simulink model "motor_discrete_velocity"  (R2015b)
settings: Solver=VariableStepAuto  StartTime=0.0  StopTime=simtime  RelTol=1e-3
values from neighbouring files (symbols this model uses):
  D = [0 0; 0 0; 0 0]    [Velocity_ctrl_HYDRAULIC.m]    (also in ex1.m = 0; position_ctrl.m = 0; velocity_ctrl.m = 0)
  d_v = 1    [ex1.m]    (also in motor_parameters.mat; position_ctrl.m; velocity_ctrl.m)
  enable_karnop = 0    [discrete_velocity.m]    (also in ex1.m = 1; motor_parameters.mat = 1; pcontrol.m; pcontrol_position.m)
  enable_sin = 0    [discrete_velocity.m]    (also in ex1.m = 1; motor_parameters.mat; pcontrol.m = 1; pcontrol_position.m = 1)
  F_c = 1e-3    (= 0.001)    [ex1.m]    (also in motor_parameters.mat; position_ctrl.m; velocity_ctrl.m)
  I = 1    [ex1.m]    (also in pcontrol.m = 0; pcontrol_position.m = 0; picontroller.m = omega1*omega2*n*Jtot*m.R/m.k; position_ctrl.m = 2)
  J = J1+J2    (= 3.6e-05)    [ex1.m]    (also in lec_example.m = 0.1; position_ctrl.m; velocity_ctrl.m)
  motor = motor_pars    [ex1.m]    (also in position_ctrl.m; velocity_ctrl.m)
  n = 5    [ex1.m]    (also in motor_parameters.mat; position_ctrl.m; velocity_ctrl.m)
  P = 0.5    [Velocity_ctrl_HYDRAULIC.m]    (also in ex1.m = 20; pcontrol.m = 8; pcontrol_position.m = 4; picontroller.m = n*(Jtot*omega1*m.R+Jtot*omega2*m.R-m.d*m.R-m.k^2)/m.k)
  sim_sin_amp = 200    [ex1.m]    (also in motor_parameters.mat = 1; pcontrol.m = 10; pcontrol_position.m = 10; pdcontroller_position.m = 10)
  sim_sin_freq = 10    [ex1.m]    (also in motor_parameters.mat = 1; pcontrol.m = 1; pcontrol_position.m = 1; pdcontroller_position.m = 1)
  sim_v = Vmax    (= 24)    [ex1.m]    (also in motor_parameters.mat; pcontrol.m = 1; pcontrol_position.m = 1; pdcontroller_position.m = 1)
  sim_zoh = 0.02    [discrete_velocity.m]    (also in pcontrol.m = 0.002; pcontrol_position.m; pdcontroller_position.m = 0.002; picontroller.m = 0.002)
  sim_zoh_sample_time = zoh_sample_time*1e-3    (= 2e-06)    [discrete_velocity.m]    (also in ex1.m = 0; motor_parameters.mat = 0; position_ctrl.m; velocity_ctrl.m)
libraries: simulink x3
settings Model: Creator=Gabriel  LastModifiedBy=Gabriel

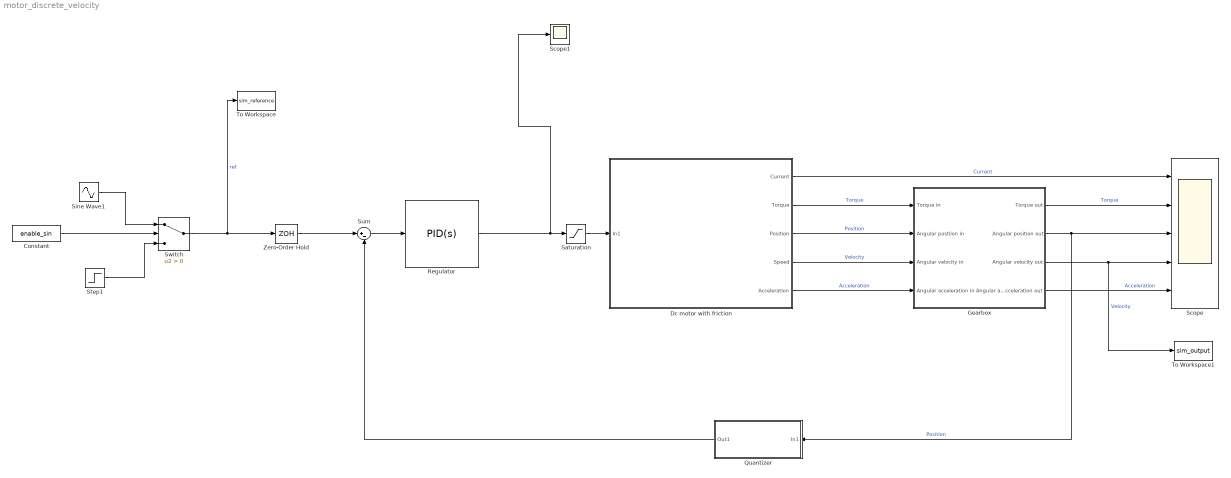
== system motor_discrete_velocity ==
  Constant : Constant  Value=enable_sin
  Dc motor with friction : Subsystem
      mask Display:
      | image('dcmotor.jpg')
      | port_label('input', 1, 'Voltage')
      | port_label('output', 1, 'Current')
      | port_label('output', 2, 'Torque')
      | port_label('output', 3, 'Position')
      | port_label('output', 4, 'Velocity')
      | port_label('output', 5, 'Acceleration')
  Gearbox : Subsystem
  "Quantizer " : Subsystem
  Regulator : simulink/Continuous/PID Controller  Controller=PID  TimeDomain=Continuous-time  SampleTime=-1  IntegratorMethod=Forward Euler  FilterMethod=Forward Euler  Form=Parallel  UseFilter=on  ControllerParametersSource=internal  P=P  I=I  D=D  N=100  InitialConditionSource=internal  InitialConditionForIntegrator=0  InitialConditionForFilter=0  ExternalReset=none  LimitOutput=off  UpperSaturationLimit=inf  LowerSaturationLimit=-inf  LinearizeAsGain=on  AntiWindupMode=none  Kb=1  TrackingMode=off  Kt=1  PParamMin=[]  PParamMax=[]  IParamMin=[]  IParamMax=[]  DParamMin=[]  DParamMax=[]  NParamMin=[]  NParamMax=[]  KbParamMin=[]  KbParamMax=[]  KtParamMin=[]  KtParamMax=[]  POutMin=[]  POutMax=[]  IOutMin=[]  IOutMax=[]  DOutMin=[]  DOutMax=[]  NOutMin=[]  NOutMax=[]  KbOutMin=[]  KbOutMax=[]  KtOutMin=[]  KtOutMax=[]  IntegratorOutMin=[]  IntegratorOutMax=[]  FilterOutMin=[]  FilterOutMax=[]  SumOutMin=[]  SumOutMax=[]  SumI1OutMin=[]  SumI1OutMax=[]  SumI2OutMin=[]  SumI2OutMax=[]  SumI3OutMin=[]  SumI3OutMax=[]  SumDOutMin=[]  SumDOutMax=[]  SaturationOutMin=[]  SaturationOutMax=[]  IntegratorContinuousStateAttributes=''  IntegratorStateMustResolveToSignalObject=off  IntegratorRTWStateStorageClass=Auto  FilterContinuousStateAttributes=''  FilterStateMustResolveToSignalObject=off  FilterRTWStateStorageClass=Auto  DifferentiatorICPrevScaledInput=0  DifferentiatorOutMin=[]  DifferentiatorOutMax=[]
  Saturation : Saturate  UpperLimit=24  LowerLimit=-24
  Scope : Scope  NumInputPorts=5
  Scope1 : Scope
  Sine Wave1 : Sin  Amplitude=sim_sin_amp  Frequency=sim_sin_freq  SampleTime=0
  Step1 : Step  Time=0  After=sim_v  SampleTime=0
  Sum : Sum  Inputs=|+-
  Switch : Switch  Criteria=u2 > Threshold
  To Workspace : ToWorkspace  VariableName=sim_reference  SaveFormat=Timeseries  SampleTime=-1
  To Workspace1 : ToWorkspace  VariableName=sim_output  SaveFormat=Timeseries  SampleTime=-1
  Zero-Order Hold : ZeroOrderHold  SampleTime=sim_zoh
  wires:
  Sum/1 -> Regulator/1
  Zero-Order Hold/1 -> Sum/1
  Step1/1 -> Switch/3
  Sine Wave1/1 -> Switch/1
  Constant/1 -> Switch/2
  Switch/1 -> Zero-Order Hold/1, To Workspace/1  "ref"
  Dc motor with friction/4(Speed) -> Gearbox/3(Angular velocity in)  "Velocity"
  Dc motor with friction/2(Torque) -> Gearbox/1(Torque in)  "Torque"
  Dc motor with friction/1(Current) -> Scope/1  "Current"
  Dc motor with friction/5(Acceleration) -> Gearbox/4(Angular acceleration in)  "Acceleration"
  Dc motor with friction/3(Position) -> Gearbox/2(Angular postiion in)  "Position"
  Gearbox/1(Torque out) -> Scope/2  "Torque"
  Gearbox/2(Angular position out) -> "Quantizer "/1(In1), Scope/3  "Position"
  Gearbox/3(Angular velocity out) -> To Workspace1/1, Scope/4  "Velocity"
  Gearbox/4(Angular acceleration out) -> Scope/5  "Acceleration"
  Regulator/1 -> Saturation/1, Scope1/1
  "Quantizer "/1(Out1) -> Sum/2
  Saturation/1 -> Dc motor with friction/1(In1)

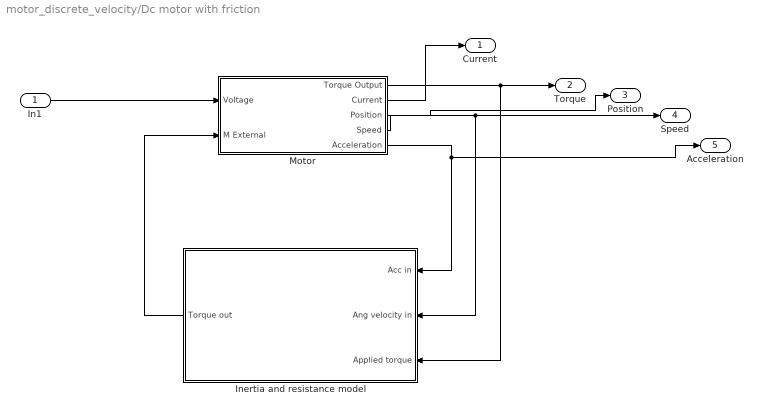
== system motor_discrete_velocity/Dc motor with friction ==
  In1 : Inport
  "Inertia and resistance model " : Subsystem
  Motor : Subsystem
  Current : Outport
  Torque : Outport  Port=2
  Position : Outport  Port=3
  Speed : Outport  Port=4
  Acceleration : Outport  Port=5
  wires:
  Motor/4(Speed) -> Speed/1, "Inertia and resistance model "/2(Ang velocity in)
  Motor/3(Position) -> Position/1
  Motor/2(Current) -> Current/1
  "Inertia and resistance model "/1(Torque out) -> Motor/2("M External ")
  Motor/1(Torque Output) -> Torque/1, "Inertia and resistance model "/3(Applied torque)
  In1/1 -> Motor/1(Voltage)
  Motor/5(Acceleration) -> "Inertia and resistance model "/1(Acc in), Acceleration/1

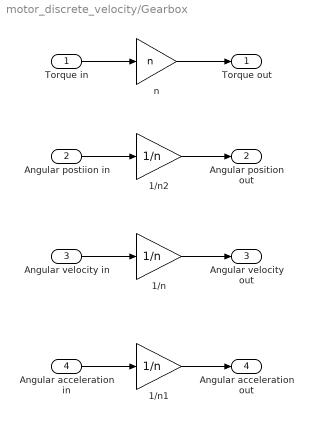
== system motor_discrete_velocity/Gearbox ==
  Torque in : Inport
  Angular postiion in : Inport  Port=2
  Angular velocity in : Inport  Port=3
  Angular acceleration in : Inport  Port=4
  1/n : Gain  Gain=1/n
  1/n1 : Gain  Gain=1/n
  1/n2 : Gain  Gain=1/n
  n : Gain  Gain=n
  Torque out : Outport
  Angular position out : Outport  Port=2
  Angular velocity out : Outport  Port=3
  Angular acceleration out : Outport  Port=4
  wires:
  1/n/1 -> Angular velocity out/1
  Angular velocity in/1 -> 1/n/1
  n/1 -> Torque out/1
  Torque in/1 -> n/1
  1/n1/1 -> Angular acceleration out/1
  Angular acceleration in/1 -> 1/n1/1
  1/n2/1 -> Angular position out/1
  Angular postiion in/1 -> 1/n2/1

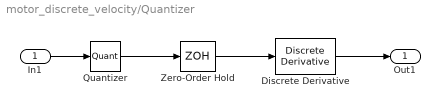
== system motor_discrete_velocity/Quantizer  ==
  In1 : Inport
  Discrete Derivative : simulink/Discrete/Discrete Derivative  gainval=1.0  ICPrevScaledInput=0.0  InputProcessing=Inherited  OutMin=[]  OutMax=[]  OutDataType=fixdt(1, 16)  OutScaling=2^-10  DoSatur=off
  Quantizer : Quantizer  QuantizationInterval=sim_quantization_interval
  Zero-Order Hold : ZeroOrderHold  SampleTime=sim_zoh_sample_time
  Out1 : Outport
  wires:
  In1/1 -> Quantizer/1
  Discrete Derivative/1 -> Out1/1
  Quantizer/1 -> Zero-Order Hold/1
  Zero-Order Hold/1 -> Discrete Derivative/1

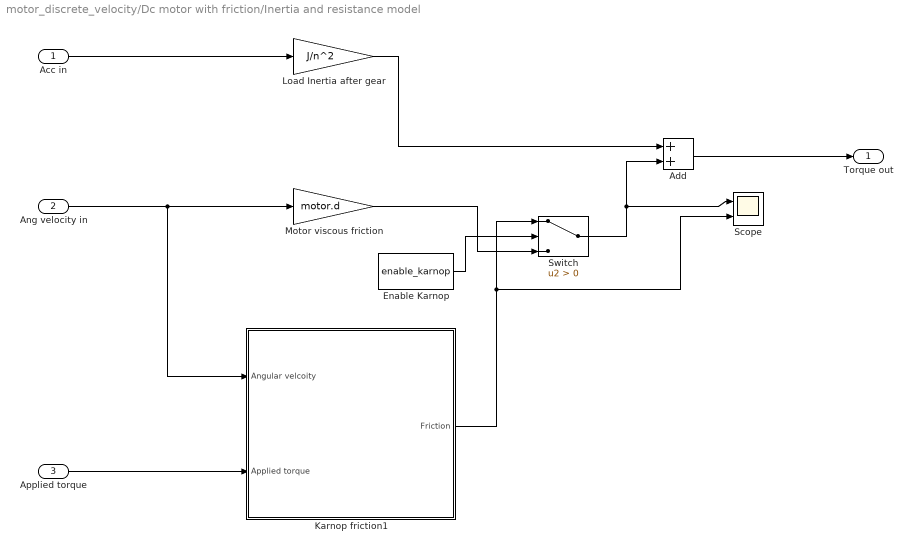
== system motor_discrete_velocity/Dc motor with friction/Inertia and resistance model  ==
  Acc in : Inport
  Ang velocity in : Inport  Port=2
  Applied torque : Inport  Port=3
  Add : Sum
  Enable Karnop : Constant  Value=enable_karnop
  Karnop friction1 : Subsystem
  Load Inertia after gear : Gain  Gain=J/n^2
  Motor viscous friction : Gain  Gain=motor.d
  Scope : Scope  NumInputPorts=2
  Switch : Switch  Criteria=u2 > Threshold
  Torque out : Outport
  wires:
  Acc in/1 -> Load Inertia after gear/1
  Add/1 -> Torque out/1
  Load Inertia after gear/1 -> Add/1
  Ang velocity in/1 -> Karnop friction1/1(Angular velcoity), Motor viscous friction/1
  Motor viscous friction/1 -> Switch/3
  Karnop friction1/1(Friction) -> Switch/1, Scope/2
  Switch/1 -> Add/2, Scope/1
  Enable Karnop/1 -> Switch/2
  Applied torque/1 -> Karnop friction1/2("Applied torque ")

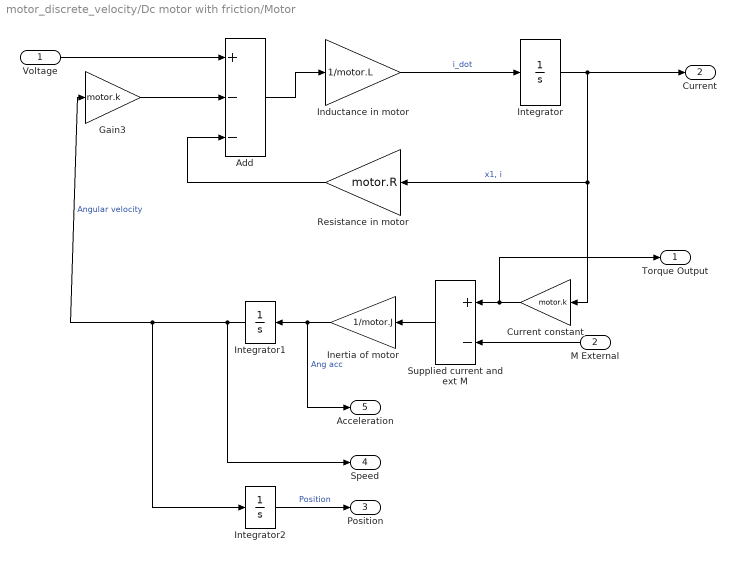
== system motor_discrete_velocity/Dc motor with friction/Motor ==
  Voltage : Inport
  "M External " : Inport  Port=2
  Add : Sum  Inputs=+--
  Current constant : Gain  Gain=motor.k
  Gain3 : Gain  Gain=motor.k
  Inductance in motor : Gain  Gain=1/motor.L
  Inertia of motor : Gain  Gain=1/motor.J
  Integrator : Integrator
  Integrator1 : Integrator
  Integrator2 : Integrator
  Resistance in motor : Gain  Gain=motor.R
  "Supplied current and ext M " : Sum  Inputs=+-
  Torque Output : Outport
  Current : Outport  Port=2
  Position : Outport  Port=3
  Speed : Outport  Port=4
  Acceleration : Outport  Port=5
  wires:
  Voltage/1 -> Add/1
  Add/1 -> Inductance in motor/1
  Inductance in motor/1 -> Integrator/1  "i_dot"
  Integrator/1 -> Current constant/1, Resistance in motor/1, Current/1  "x1, i"
  Resistance in motor/1 -> Add/3
  Gain3/1 -> Add/2
  Integrator1/1 -> Speed/1, Integrator2/1, Gain3/1  "Angular velocity"
  "Supplied current and ext M "/1 -> Inertia of motor/1
  Inertia of motor/1 -> Acceleration/1, Integrator1/1  "Ang acc"
  Current constant/1 -> Torque Output/1, "Supplied current and ext M "/1
  "M External "/1 -> "Supplied current and ext M "/2
  Integrator2/1 -> Position/1  "Position"

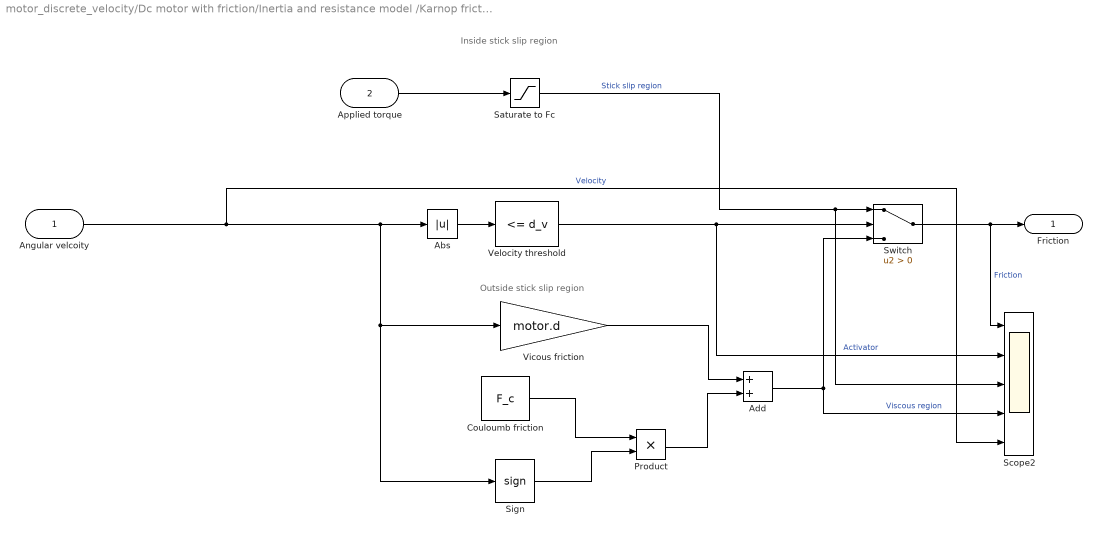
== system motor_discrete_velocity/Dc motor with friction/Inertia and resistance model /Karnop friction1 ==
  note: Inside stick slip region
  note: Outside stick slip region
  Angular velcoity : Inport
  "Applied torque " : Inport  Port=2
  Abs : Abs
  Add : Sum
  Couloumb friction : Constant  Value=F_c
  Product : Product
  Saturate to Fc : Saturate  UpperLimit=F_c  LowerLimit=-F_c
  Scope2 : Scope  NumInputPorts=5
  Sign : Signum
  Switch : Switch  Criteria=u2 > Threshold
  "Velocity threshold " : simulink/Logic and Bit Operations/Compare To Constant  relop=<=  const=d_v  OutDataTypeStr=uint8
  Vicous friction : Gain  Gain=motor.d
  Friction : Outport
  wires:
  Saturate to Fc/1 -> Scope2/3, Switch/1  "Stick slip region"
  Switch/1 -> Scope2/1, Friction/1  "Friction"
  Angular velcoity/1 -> Scope2/5, Abs/1, Vicous friction/1, Sign/1  "Velocity"
  "Velocity threshold "/1 -> Scope2/2, Switch/2  "Activator"
  Abs/1 -> "Velocity threshold "/1
  Product/1 -> Add/2
  Vicous friction/1 -> Add/1
  Couloumb friction/1 -> Product/1
  Sign/1 -> Product/2
  "Applied torque "/1 -> Saturate to Fc/1
  Add/1 -> Switch/3, Scope2/4  "Viscous region"
